simulink model "RosConnector"  (R2020a)
settings: Solver=VariableStepAuto  StartTime=0.0  StopTime=inf  RelTol=1e-3
libraries: robotlib x9, simulink x3
settings Model: Creator=user  LastModifiedBy=user

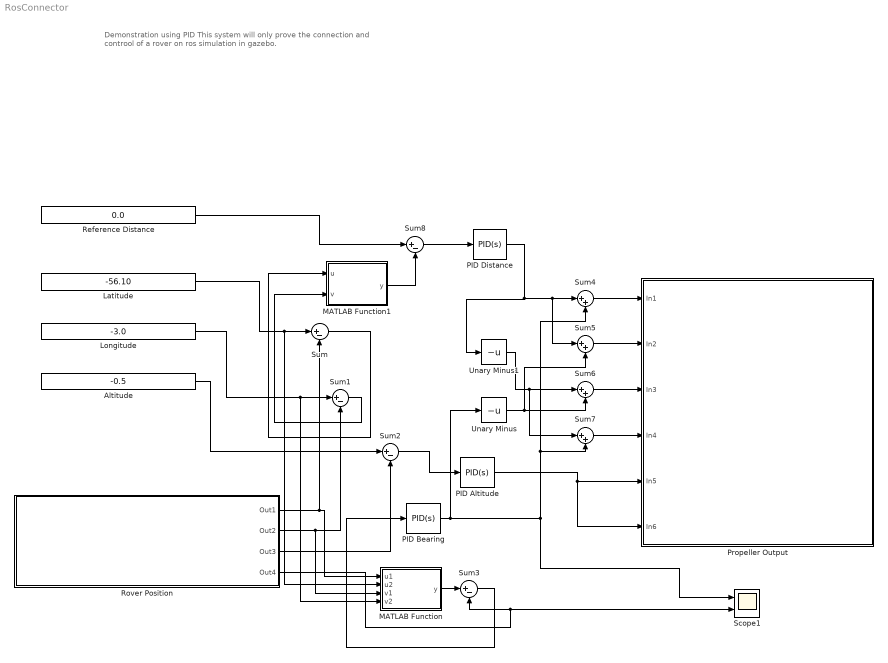
== system RosConnector ==
  note: Demonstration using PID
      |
      | This system will only prove the connection and controol of a rover on ros simulation in gazebo.
  Altitude : Constant  Value=-0.5
  Latitude : Constant  Value=-56.10
  Longitude : Constant  Value=-3.0
  MATLAB Function : MATLAB Function  TreatAsAtomicUnit=on
  MATLAB Function1 : MATLAB Function  TreatAsAtomicUnit=on
  PID Altitude : simulink/Continuous/PID Controller  Controller=PID  Form=Parallel  TimeDomain=Continuous-time  UseExternalTs=off  SampleTime=-1  IntegratorMethod=Forward Euler  FilterMethod=Forward Euler  ControllerParametersSource=internal  P=1  I=1  D=0  UseFilter=on  N=100  TunerSelectOption=Transfer Function Based (PID Tuner App)  InitialConditionSource=internal  InitialConditionForIntegrator=0  InitialConditionForFilter=0  DifferentiatorICPrevScaledInput=0  ExternalReset=none  TrackingMode=off  Kt=1  LimitOutput=off  UpperSaturationLimit=inf  LowerSaturationLimit=-inf  LinearizeAsGain=on  AntiWindupMode=none  Kb=1  POutMin=[]  POutMax=[]  IOutMin=[]  IOutMax=[]  DOutMin=[]  DOutMax=[]  NOutMin=[]  NOutMax=[]  SumOutMin=[]  SumOutMax=[]  SaturationOutMin=[]  SaturationOutMax=[]  PParamMin=[]  PParamMax=[]  IParamMin=[]  IParamMax=[]  DParamMin=[]  DParamMax=[]  NParamMin=[]  NParamMax=[]  KbParamMin=[]  KbParamMax=[]  KtParamMin=[]  KtParamMax=[]  KbOutMin=[]  KbOutMax=[]  KtOutMin=[]  KtOutMax=[]  IntegratorOutMin=[]  IntegratorOutMax=[]  FilterOutMin=[]  FilterOutMax=[]  SumI1OutMin=[]  SumI1OutMax=[]  SumI2OutMin=[]  SumI2OutMax=[]  SumI3OutMin=[]  SumI3OutMax=[]  SumI4OutMin=[]  SumI4OutMax=[]  SumDOutMin=[]  SumDOutMax=[]  DifferentiatorOutMin=[]  DifferentiatorOutMax=[]  FilterDiffOutCoefMin=[]  FilterDiffOutCoefMax=[]  ReciprocalOutMin=[]  ReciprocalOutMax=[]  SumDenOutMin=[]  SumDenOutMax=[]  SumNumOutMin=[]  SumNumOutMax=[]  DivideOutMin=[]  DivideOutMax=[]  UdiffTsProdOutMin=[]  UdiffTsProdOutMax=[]  NTsProdOutMin=[]  NTsProdOutMax=[]  UintegralTsProdOutMin=[]  UintegralTsProdOutMax=[]  UngainTsProdOutMin=[]  UngainTsProdOutMax=[]  IntegratorContinuousStateAttributes=''  IntegratorStateMustResolveToSignalObject=off  IntegratorRTWStateStorageClass=Auto  FilterContinuousStateAttributes=''  FilterStateMustResolveToSignalObject=off  FilterRTWStateStorageClass=Auto  ParallelPVariant=InternalParameters  IdealPVariant=Disabled  IVariant=InternalParameters  DVariant=InternalParameters  IntegratorVariant=Continuous  SatVariant=Disabled  AWVariant=Passthrough  PCopyVariant=Disabled  TRVariant=Disabled  FdbkBlocksVariant=Forward  IdealPFdbkVariant=Disabled  SatFdbkVariant=Disabled  DerivativeFilterVariant=ContFilter  NVariant=InternalParameters  NCopyVariant=Disabled  FilterICVariant=InternalICsFilter  IntegratorICVariant=InternalICs  ExternalResetVariant=Disabled  TRSumVariant=Passthrough  SumFdbkVariant=Disabled  SumVariant=Sum_PID  TsampFilterVariant=InternalTs  TsampNgainVariant=Passthrough  TsampIntegralVariant=Passthrough
  PID Bearing : simulink/Continuous/PID Controller  Controller=PID  Form=Parallel  TimeDomain=Continuous-time  UseExternalTs=off  SampleTime=-1  IntegratorMethod=Forward Euler  FilterMethod=Forward Euler  ControllerParametersSource=internal  P=1  I=1  D=0  UseFilter=on  N=100  TunerSelectOption=Transfer Function Based (PID Tuner App)  InitialConditionSource=internal  InitialConditionForIntegrator=0  InitialConditionForFilter=0  DifferentiatorICPrevScaledInput=0  ExternalReset=none  TrackingMode=off  Kt=1  LimitOutput=off  UpperSaturationLimit=inf  LowerSaturationLimit=-inf  LinearizeAsGain=on  AntiWindupMode=none  Kb=1  POutMin=[]  POutMax=[]  IOutMin=[]  IOutMax=[]  DOutMin=[]  DOutMax=[]  NOutMin=[]  NOutMax=[]  SumOutMin=[]  SumOutMax=[]  SaturationOutMin=[]  SaturationOutMax=[]  PParamMin=[]  PParamMax=[]  IParamMin=[]  IParamMax=[]  DParamMin=[]  DParamMax=[]  NParamMin=[]  NParamMax=[]  KbParamMin=[]  KbParamMax=[]  KtParamMin=[]  KtParamMax=[]  KbOutMin=[]  KbOutMax=[]  KtOutMin=[]  KtOutMax=[]  IntegratorOutMin=[]  IntegratorOutMax=[]  FilterOutMin=[]  FilterOutMax=[]  SumI1OutMin=[]  SumI1OutMax=[]  SumI2OutMin=[]  SumI2OutMax=[]  SumI3OutMin=[]  SumI3OutMax=[]  SumI4OutMin=[]  SumI4OutMax=[]  SumDOutMin=[]  SumDOutMax=[]  DifferentiatorOutMin=[]  DifferentiatorOutMax=[]  FilterDiffOutCoefMin=[]  FilterDiffOutCoefMax=[]  ReciprocalOutMin=[]  ReciprocalOutMax=[]  SumDenOutMin=[]  SumDenOutMax=[]  SumNumOutMin=[]  SumNumOutMax=[]  DivideOutMin=[]  DivideOutMax=[]  UdiffTsProdOutMin=[]  UdiffTsProdOutMax=[]  NTsProdOutMin=[]  NTsProdOutMax=[]  UintegralTsProdOutMin=[]  UintegralTsProdOutMax=[]  UngainTsProdOutMin=[]  UngainTsProdOutMax=[]  IntegratorContinuousStateAttributes=''  IntegratorStateMustResolveToSignalObject=off  IntegratorRTWStateStorageClass=Auto  FilterContinuousStateAttributes=''  FilterStateMustResolveToSignalObject=off  FilterRTWStateStorageClass=Auto  ParallelPVariant=InternalParameters  IdealPVariant=Disabled  IVariant=InternalParameters  DVariant=InternalParameters  IntegratorVariant=Continuous  SatVariant=Disabled  AWVariant=Passthrough  PCopyVariant=Disabled  TRVariant=Disabled  FdbkBlocksVariant=Forward  IdealPFdbkVariant=Disabled  SatFdbkVariant=Disabled  DerivativeFilterVariant=ContFilter  NVariant=InternalParameters  NCopyVariant=Disabled  FilterICVariant=InternalICsFilter  IntegratorICVariant=InternalICs  ExternalResetVariant=Disabled  TRSumVariant=Passthrough  SumFdbkVariant=Disabled  SumVariant=Sum_PID  TsampFilterVariant=InternalTs  TsampNgainVariant=Passthrough  TsampIntegralVariant=Passthrough
  PID Distance : simulink/Continuous/PID Controller  Controller=PID  Form=Parallel  TimeDomain=Continuous-time  UseExternalTs=off  SampleTime=-1  IntegratorMethod=Forward Euler  FilterMethod=Forward Euler  ControllerParametersSource=internal  P=1  I=1  D=0  UseFilter=on  N=100  TunerSelectOption=Transfer Function Based (PID Tuner App)  InitialConditionSource=internal  InitialConditionForIntegrator=0  InitialConditionForFilter=0  DifferentiatorICPrevScaledInput=0  ExternalReset=none  TrackingMode=off  Kt=1  LimitOutput=off  UpperSaturationLimit=inf  LowerSaturationLimit=-inf  LinearizeAsGain=on  AntiWindupMode=none  Kb=1  POutMin=[]  POutMax=[]  IOutMin=[]  IOutMax=[]  DOutMin=[]  DOutMax=[]  NOutMin=[]  NOutMax=[]  SumOutMin=[]  SumOutMax=[]  SaturationOutMin=[]  SaturationOutMax=[]  PParamMin=[]  PParamMax=[]  IParamMin=[]  IParamMax=[]  DParamMin=[]  DParamMax=[]  NParamMin=[]  NParamMax=[]  KbParamMin=[]  KbParamMax=[]  KtParamMin=[]  KtParamMax=[]  KbOutMin=[]  KbOutMax=[]  KtOutMin=[]  KtOutMax=[]  IntegratorOutMin=[]  IntegratorOutMax=[]  FilterOutMin=[]  FilterOutMax=[]  SumI1OutMin=[]  SumI1OutMax=[]  SumI2OutMin=[]  SumI2OutMax=[]  SumI3OutMin=[]  SumI3OutMax=[]  SumI4OutMin=[]  SumI4OutMax=[]  SumDOutMin=[]  SumDOutMax=[]  DifferentiatorOutMin=[]  DifferentiatorOutMax=[]  FilterDiffOutCoefMin=[]  FilterDiffOutCoefMax=[]  ReciprocalOutMin=[]  ReciprocalOutMax=[]  SumDenOutMin=[]  SumDenOutMax=[]  SumNumOutMin=[]  SumNumOutMax=[]  DivideOutMin=[]  DivideOutMax=[]  UdiffTsProdOutMin=[]  UdiffTsProdOutMax=[]  NTsProdOutMin=[]  NTsProdOutMax=[]  UintegralTsProdOutMin=[]  UintegralTsProdOutMax=[]  UngainTsProdOutMin=[]  UngainTsProdOutMax=[]  IntegratorContinuousStateAttributes=''  IntegratorStateMustResolveToSignalObject=off  IntegratorRTWStateStorageClass=Auto  FilterContinuousStateAttributes=''  FilterStateMustResolveToSignalObject=off  FilterRTWStateStorageClass=Auto  ParallelPVariant=InternalParameters  IdealPVariant=Disabled  IVariant=InternalParameters  DVariant=InternalParameters  IntegratorVariant=Continuous  SatVariant=Disabled  AWVariant=Passthrough  PCopyVariant=Disabled  TRVariant=Disabled  FdbkBlocksVariant=Forward  IdealPFdbkVariant=Disabled  SatFdbkVariant=Disabled  DerivativeFilterVariant=ContFilter  NVariant=InternalParameters  NCopyVariant=Disabled  FilterICVariant=InternalICsFilter  IntegratorICVariant=InternalICs  ExternalResetVariant=Disabled  TRSumVariant=Passthrough  SumFdbkVariant=Disabled  SumVariant=Sum_PID  TsampFilterVariant=InternalTs  TsampNgainVariant=Passthrough  TsampIntegralVariant=Passthrough
  Propeller Output : Subsystem
  Reference Distance : Constant  Value=0.0
  Rover Position : Subsystem
  Scope1 : Scope  NumInputPorts=2
  Sum{,1..3,8} (5 alike) : Sum  Inputs=|+-
  Sum{4..7} (4 alike) : Sum  Inputs=|++
  Unary Minus : UnaryMinus
  Unary Minus1 : UnaryMinus
  wires:
  Latitude/1 -> MATLAB Function/2(u2), Sum/1
  Rover Position/1(Out1) -> MATLAB Function/1(u1), Sum/2
  Longitude/1 -> MATLAB Function/4(v2), Sum1/1
  Rover Position/2(Out2) -> MATLAB Function/3(v1), Sum1/2
  Altitude/1 -> Sum2/1
  Rover Position/3(Out3) -> Sum2/2
  Sum2/1 -> PID Altitude/1
  PID Altitude/1 -> Propeller Output/6(In6), Propeller Output/5(In5)
  PID Bearing/1 -> Unary Minus/1, Sum7/2, Sum4/2, Scope1/1
  Rover Position/4(Out4) -> Scope1/2, Sum3/2
  Sum3/1 -> PID Bearing/1
  MATLAB Function/1(y) -> Sum3/1
  Sum4/1 -> Propeller Output/1(In1)
  Sum7/1 -> Propeller Output/4(In4)
  Sum6/1 -> Propeller Output/3(In3)
  Sum5/1 -> Propeller Output/2(In2)
  Unary Minus/1 -> Sum5/2, Sum6/2
  Sum1/1 -> MATLAB Function1/2(v)
  Sum/1 -> MATLAB Function1/1(u)
  MATLAB Function1/1(y) -> Sum8/2
  Reference Distance/1 -> Sum8/1
  Unary Minus1/1 -> Sum7/1, Sum6/1
  Sum8/1 -> PID Distance/1
  PID Distance/1 -> Sum5/1, Sum4/1, Unary Minus1/1

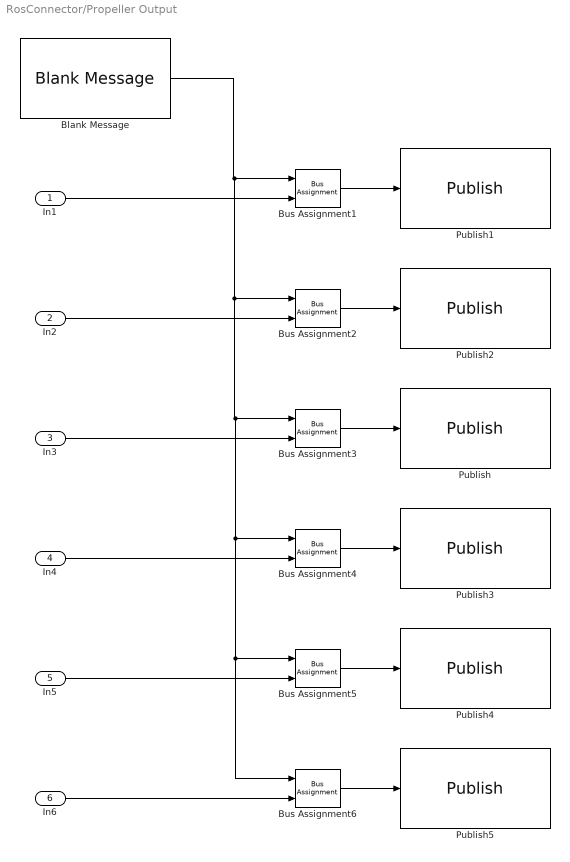
== system RosConnector/Propeller Output ==
  In1 : Inport
  In2 : Inport  Port=2
  In3 : Inport  Port=3
  In4 : Inport  Port=4
  In5 : Inport  Port=5
  In6 : Inport  Port=6
  Blank Message : robotlib/Blank Message  messageClass=Message  entityType=uuv_gazebo_ros_plugins_msgs/FloatStamped  messageType=uuv_gazebo_ros_plugins_msgs/FloatStamped  SampleTime=inf
  Bus Assignment{1..6} (6 alike) : BusAssignment  AssignedSignals=Data
  Publish : robotlib/Publish  topicSource=Select from ROS network  topic=/bluerov2/thrusters/2/input  messageType=uuv_gazebo_ros_plugins_msgs/FloatStamped  messageQueueLength=1
  Publish1 : robotlib/Publish  topicSource=Select from ROS network  topic=/bluerov2/thrusters/0/input  messageType=uuv_gazebo_ros_plugins_msgs/FloatStamped  messageQueueLength=1
  Publish2 : robotlib/Publish  topicSource=Select from ROS network  topic=/bluerov2/thrusters/1/input  messageType=uuv_gazebo_ros_plugins_msgs/FloatStamped  messageQueueLength=1
  Publish3 : robotlib/Publish  topicSource=Select from ROS network  topic=/bluerov2/thrusters/3/input  messageType=uuv_gazebo_ros_plugins_msgs/FloatStamped  messageQueueLength=1
  Publish4 : robotlib/Publish  topicSource=Select from ROS network  topic=/bluerov2/thrusters/4/input  messageType=uuv_gazebo_ros_plugins_msgs/FloatStamped  messageQueueLength=1
  Publish5 : robotlib/Publish  topicSource=Select from ROS network  topic=/bluerov2/thrusters/5/input  messageType=uuv_gazebo_ros_plugins_msgs/FloatStamped  messageQueueLength=1
  wires:
  Bus Assignment5/1 -> Publish4/1
  Bus Assignment4/1 -> Publish3/1
  Bus Assignment3/1 -> Publish/1
  Bus Assignment2/1 -> Publish2/1
  Bus Assignment1/1 -> Publish1/1
  Bus Assignment6/1 -> Publish5/1
  Blank Message/1 -> Bus Assignment6/1, Bus Assignment5/1, Bus Assignment4/1, Bus Assignment3/1, Bus Assignment2/1, Bus Assignment1/1
  In1/1 -> Bus Assignment1/2
  In2/1 -> Bus Assignment2/2
  In3/1 -> Bus Assignment3/2
  In4/1 -> Bus Assignment4/2
  In5/1 -> Bus Assignment5/2
  In6/1 -> Bus Assignment6/2

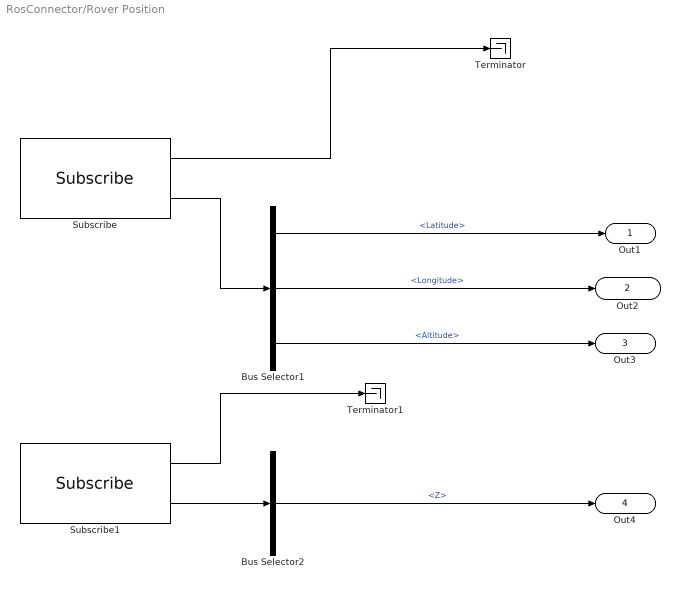
== system RosConnector/Rover Position ==
  Bus Selector1 : BusSelector  OutputSignals=Latitude,Longitude,Altitude
  Bus Selector2 : BusSelector  OutputSignals=Orientation.Z
  Subscribe : robotlib/Subscribe  topicSource=Select from ROS network  topic=/bluerov2/gps  messageType=sensor_msgs/NavSatFix  sampleTime=-1  messageQueueLength=1
  Subscribe1 : robotlib/Subscribe  topicSource=Select from ROS network  topic=/bluerov2/imu  messageType=sensor_msgs/Imu  sampleTime=-1  messageQueueLength=1
  Terminator : Terminator
  Terminator1 : Terminator
  Out1 : Outport
  Out2 : Outport  Port=2
  Out3 : Outport  Port=3
  Out4 : Outport  Port=4
  wires:
  Subscribe/1 -> Terminator/1
  Bus Selector1/1 -> Out1/1  "<Latitude>"
  Subscribe/2 -> Bus Selector1/1
  Bus Selector1/2 -> Out2/1  "<Longitude>"
  Bus Selector1/3 -> Out3/1  "<Altitude>"
  Subscribe1/2 -> Bus Selector2/1
  Subscribe1/1 -> Terminator1/1
  Bus Selector2/1 -> Out4/1  "<Z>"

== matlab function RosConnector/MATLAB Function1 ==
  data: u input; y output; v input
function y = fcn(u,v)

% Using pythagoras theorem to find distance between actual and required.
y = sqrt((u^2)+(v^2));

== matlab function RosConnector/MATLAB Function ==
  data: u1 input; y output; u2 input; v1 input; v2 input
function y = fcn(u1,u2,v1,v2)

y = pi/2 - atan((v2-v1)-(u2-u1));
